simulink model "sim_task_1"  (R2024a)
settings: Solver=FixedStepAuto  StartTime=0.0  StopTime=5.0  FixedStep=1e-3  RelTol=1e-3
settings Model: Creator=alexe  LastModifiedBy=alexe

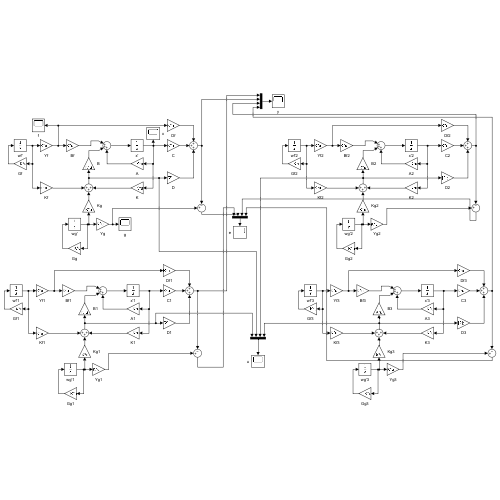
[thumbnail: Simulink's stored preview of the top-level diagram]
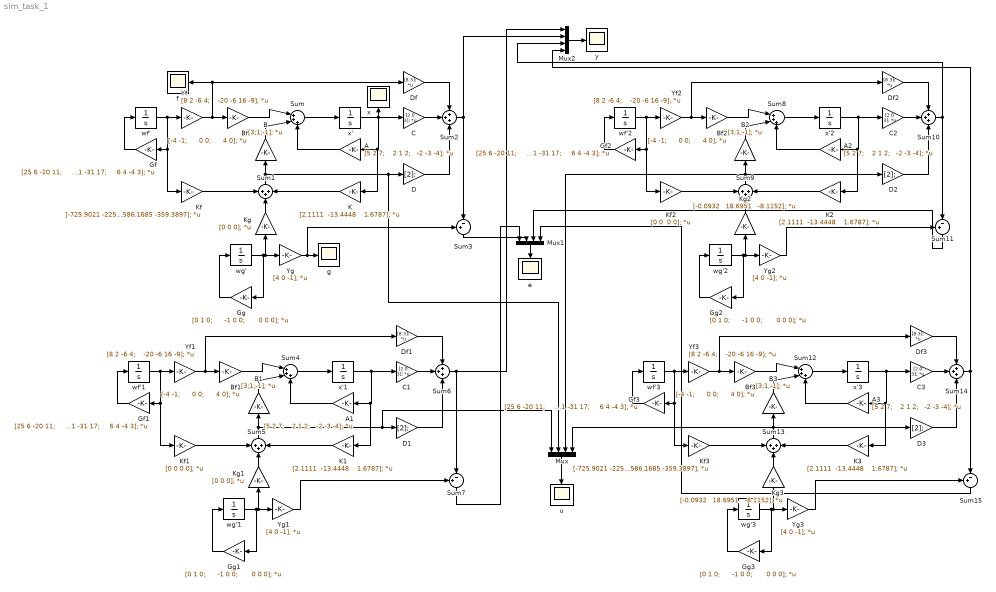
== system sim_task_1 ==
  A : Gain  Gain=|  Multiplication=Matrix(K*u)
      | [5 2 7;
      |    2 1 2;
      |   -2 -3 -4];
  A1 : Gain  Gain=|  Multiplication=Matrix(K*u)
      | [5 2 7;
      |    2 1 2;
      |   -2 -3 -4];
  A2 : Gain  Gain=|  Multiplication=Matrix(K*u)
      | [5 2 7;
      |    2 1 2;
      |   -2 -3 -4];
  A3 : Gain  Gain=|  Multiplication=Matrix(K*u)
      | [5 2 7;
      |    2 1 2;
      |   -2 -3 -4];
  B{,1..3} (4 alike) : Gain  Gain=[3;1;-1];  Multiplication=Matrix(K*u)
  Bf : Gain  Gain=|  Multiplication=Matrix(K*u)
      | [-4 -1;
      |      0 0;
      |      4 0];
  Bf1 : Gain  Gain=|  Multiplication=Matrix(K*u)
      | [-4 -1;
      |      0 0;
      |      4 0];
  Bf2 : Gain  Gain=|  Multiplication=Matrix(K*u)
      | [-4 -1;
      |      0 0;
      |      4 0];
  Bf3 : Gain  Gain=|  Multiplication=Matrix(K*u)
      | [-4 -1;
      |      0 0;
      |      4 0];
  C{,1..3} (4 alike) : Gain  Gain=[2 0 3];  Multiplication=Matrix(K*u)
  D{,1..3} (4 alike) : Gain  Gain=[2];
  Df{,1..3} (4 alike) : Gain  Gain=[8 3];  Multiplication=Matrix(K*u)
  Gf : Gain  Gain=|  Multiplication=Matrix(K*u)
      | [25 6 -20 11;
      |     14 3 -10 4;
      |     40 11 -31 17;
      |     6 4 -4 3];
  Gf1 : Gain  Gain=|  Multiplication=Matrix(K*u)
      | [25 6 -20 11;
      |     14 3 -10 4;
      |     40 11 -31 17;
      |     6 4 -4 3];
  Gf2 : Gain  Gain=|  Multiplication=Matrix(K*u)
      | [25 6 -20 11;
      |     14 3 -10 4;
      |     40 11 -31 17;
      |     6 4 -4 3];
  Gf3 : Gain  Gain=|  Multiplication=Matrix(K*u)
      | [25 6 -20 11;
      |     14 3 -10 4;
      |     40 11 -31 17;
      |     6 4 -4 3];
  Gg : Gain  Gain=|  Multiplication=Matrix(K*u)
      | [0 1 0;
      |      -1 0 0;
      |       0 0 0];
  Gg1 : Gain  Gain=|  Multiplication=Matrix(K*u)
      | [0 1 0;
      |      -1 0 0;
      |       0 0 0];
  Gg2 : Gain  Gain=|  Multiplication=Matrix(K*u)
      | [0 1 0;
      |      -1 0 0;
      |       0 0 0];
  Gg3 : Gain  Gain=|  Multiplication=Matrix(K*u)
      | [0 1 0;
      |      -1 0 0;
      |       0 0 0];
  K{,1..3} (4 alike) : Gain  Gain="[2.1111  -13.4448    1.6787];"  Multiplication=Matrix(K*u)
  Kf : Gain  Gain="[-725.9021 -225.1491  586.1685 -359.3897];"  Multiplication=Matrix(K*u)
  Kf1 : Gain  Gain=[0 0 0 0];  Multiplication=Matrix(K*u)
  Kf2 : Gain  Gain="[0 0  0 0];"  Multiplication=Matrix(K*u)
  Kf3 : Gain  Gain="[-725.9021 -225.1491  586.1685 -359.3897];"  Multiplication=Matrix(K*u)
  Kg : Gain  Gain=[0 0 0];  Multiplication=Matrix(K*u)
  Kg1 : Gain  Gain=[0 0 0];  Multiplication=Matrix(K*u)
  Kg2 : Gain  Gain="[-0.0932   18.6951   -8.1152];"  Multiplication=Matrix(K*u)
  Kg3 : Gain  Gain="[-0.0932   18.6951   -8.1152];"  Multiplication=Matrix(K*u)
  Mux : Mux
  Mux1 : Mux
  Mux2 : Mux
  Sum{,4,8,12} (4 alike) : Sum  Inputs=|+++
  Sum{1..2,5..6,9..10,13..14} (8 alike) : Sum  Inputs=+++
  Sum{3,7,11,15} (4 alike) : Sum  Inputs=+-|
  Yf : Gain  Gain=|  Multiplication=Matrix(K*u)
      | [8 2 -6 4;
      |    -20 -6 16 -9];
  Yf1 : Gain  Gain=|  Multiplication=Matrix(K*u)
      | [8 2 -6 4;
      |    -20 -6 16 -9];
  Yf2 : Gain  Gain=|  Multiplication=Matrix(K*u)
      | [8 2 -6 4;
      |    -20 -6 16 -9];
  Yf3 : Gain  Gain=|  Multiplication=Matrix(K*u)
      | [8 2 -6 4;
      |    -20 -6 16 -9];
  Yg{,1..3} (4 alike) : Gain  Gain=[4 0 -1];  Multiplication=Matrix(K*u)
  e : Scope
  f : Scope
  g : Scope
  u : Scope
  wf'{,1..3} (4 alike) : Integrator  InitialCondition=[1;1;1;1];
  wg'{,1..3} (4 alike) : Integrator  InitialCondition=[0;1;1];
  x : Scope
  x'{,1..3} (4 alike) : Integrator  InitialCondition=[0;0;0];
  y : Scope
  wires:
  wf'/1 -> Kf/1, Gf/1, Yf/1
  Gf/1 -> wf'/1
  A/1 -> Sum/3
  B/1 -> Sum/2
  Sum/1 -> x'/1
  x'/1 -> x/1, C/1, K/1, A/1
  Yf/1 -> f/1, Df/1, Bf/1
  Bf/1 -> Sum/1
  wg'/1 -> Gg/1, Kg/1, Yg/1
  Gg/1 -> wg'/1
  Yg/1 -> g/1, Sum3/1
  Kg/1 -> Sum1/2
  Kf/1 -> Sum1/1
  K/1 -> Sum1/3
  Sum1/1 -> Mux/2, D/1, B/1
  Df/1 -> Sum2/1
  C/1 -> Sum2/2
  D/1 -> Sum2/3
  Sum2/1 -> Mux2/2, Sum3/2
  Sum3/1 -> Mux1/2
  K1/1 -> Sum5/3
  D1/1 -> Sum6/3
  Gg1/1 -> wg'1/1
  Kg1/1 -> Sum5/2
  C1/1 -> Sum6/2
  Sum4/1 -> x'1/1
  A1/1 -> Sum4/3
  B1/1 -> Sum4/2
  Sum5/1 -> Mux/1, D1/1, B1/1
  Gf1/1 -> wf'1/1
  wg'1/1 -> Gg1/1, Kg1/1, Yg1/1
  Kf1/1 -> Sum5/1
  Sum6/1 -> Mux2/1, Sum7/2
  wf'1/1 -> Kf1/1, Gf1/1, Yf1/1
  Yf1/1 -> Df1/1, Bf1/1
  Sum7/1 -> Mux1/1
  Df1/1 -> Sum6/1
  Yg1/1 -> Sum7/1
  x'1/1 -> C1/1, K1/1, A1/1
  Bf1/1 -> Sum4/1
  K2/1 -> Sum9/3
  D2/1 -> Sum10/3
  Gg2/1 -> wg'2/1
  Kg2/1 -> Sum9/2
  C2/1 -> Sum10/2
  Sum8/1 -> x'2/1
  A2/1 -> Sum8/3
  B2/1 -> Sum8/2
  Sum9/1 -> Mux/3, D2/1, B2/1
  Gf2/1 -> wf'2/1
  wg'2/1 -> Gg2/1, Kg2/1, Yg2/1
  Kf2/1 -> Sum9/1
  Sum10/1 -> Mux2/3, Sum11/2
  wf'2/1 -> Kf2/1, Gf2/1, Yf2/1
  Yf2/1 -> Df2/1, Bf2/1
  Df2/1 -> Sum10/1
  Yg2/1 -> Sum11/1
  x'2/1 -> C2/1, K2/1, A2/1
  Bf2/1 -> Sum8/1
  K3/1 -> Sum13/3
  D3/1 -> Sum14/3
  Gg3/1 -> wg'3/1
  Kg3/1 -> Sum13/2
  C3/1 -> Sum14/2
  Sum12/1 -> x'3/1
  A3/1 -> Sum12/3
  B3/1 -> Sum12/2
  Sum13/1 -> Mux/4, D3/1, B3/1
  Gf3/1 -> wf'3/1
  wg'3/1 -> Gg3/1, Kg3/1, Yg3/1
  Kf3/1 -> Sum13/1
  Sum14/1 -> Mux2/4, Sum15/2
  wf'3/1 -> Kf3/1, Gf3/1, Yf3/1
  Yf3/1 -> Df3/1, Bf3/1
  Sum15/1 -> Mux1/4
  Df3/1 -> Sum14/1
  Yg3/1 -> Sum15/1
  x'3/1 -> C3/1, K3/1, A3/1
  Bf3/1 -> Sum12/1
  Mux/1 -> u/1
  Sum11/1 -> Mux1/3
  Mux1/1 -> e/1
  Mux2/1 -> y/1
